simulink model "Q3"  (R2020b)
settings: Solver=VariableStepAuto  StartTime=0.0  StopTime=500  RelTol=1e-3
model workspace (MATLAB code in the model file):
  | K = -1.2;
  | alpha = 0.4;
  | D1 = 30;
  | D2 = 45;
  | tau = 40;
libraries: cstblocks x2
settings Model: Creator=HP  LastModifiedBy=HP

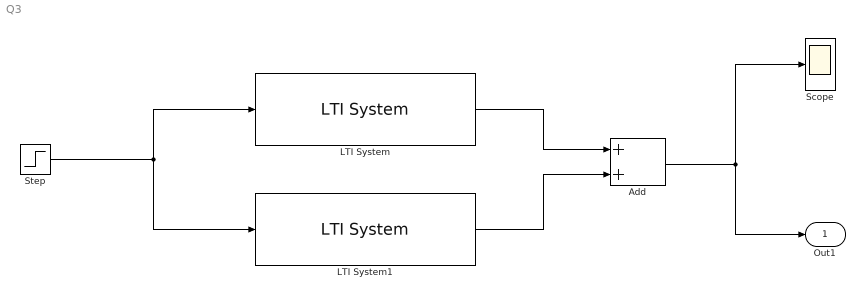
== system Q3 ==
  Add : Sum
  LTI System : cstblocks/LTI System  sys=tf(K,[tau 1],'InputDelay',D1)  IC=[]
  LTI System1 : cstblocks/LTI System  sys=tf(K*alpha,[tau 1],'InputDelay',D2+D1)  IC=[]
  Scope : Scope
  Step : Step  SampleTime=0
  Out1 : Outport
  wires:
  Step/1 -> LTI System1/1, LTI System/1
  LTI System/1 -> Add/1
  LTI System1/1 -> Add/2
  Add/1 -> Scope/1, Out1/1
